simulink library "DirectK_Lib"  (R2014a)
settings: Solver=ode45  StartTime=0.0  StopTime=10  RelTol=1e-3
settings Model: Creator=Cat  LastModifiedBy=Cat

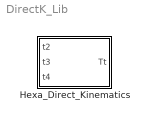
== system DirectK_Lib ==
  Hexa_Direct_Kinematics : MATLAB Function  TreatAsAtomicUnit=on

== matlab function DirectK_Lib/Hexa_Direct_Kinematics ==
  data: t2 input; Tt output; t3 input; t4 input
function Tt = Hexa_Direct_Kinematics(t2,t3,t4)
%#codegen

%    This function was generated by the Symbolic Math Toolbox version 6.0.
%    29-Sep-2015 02:51:10

t5 = t3-t4;
t6 = sin(t2);
t7 = t6.*(1.0./2.0);
t8 = sqrt(3.0);
t9 = cos(t2);
t17 = t8.*t9.*(1.0./2.0);
t10 = t7-t17;
t11 = cos(t5);
t12 = t8.*t9.*(2.0./5.0);
t13 = t9.*(1.0./2.0);
t14 = t6.*t8.*(1.0./2.0);
t15 = t13+t14;
t16 = sin(t5);
t18 = cos(t3);
t19 = t9.*(2.0./5.0);
t20 = t6.*t8.*(2.0./5.0);
t21 = t19+t20;
Tt = reshape([-t10.*t11,t11.*t15,-t16,0.0,-t10.*t16,t15.*t16,t11,0.0,t15,t10,0.0,0.0,t6.*(-2.0./5.0)+t8.*(2.0./5.0)+t12-t11.*(t6.*(2.0./5.0)-t12)-t18.*(t6-t8.*t9).*(2.0./5.0),t19+t20+t11.*t21+t18.*t21+2.0./5.0,t16.*(-4.0./5.0)-sin(t3).*(4.0./5.0),1.0],[4, 4]);
